simulink model "controller_PRM_BFS_smooth"  (R2023b)
settings: Solver=VariableStepAuto  StartTime=0.0  StopTime=200  RelTol=1e-3
StopFcn:
  | %plot_trajectory(out.x.Data(:,1), out.y.Data(:,1), 'x [m]', 'y [m]', fullfile('C:\Users\paolo\OneDrive - MSFT\Documenti\Personali\Scuola\università\magistrale\2° ANNO\Secondo Semestre\FSR\Project\Software\Images\Paper\Chapter_4_simulation\smooth\simulink', 'current_trajectory.pdf'));
  | %plot_trajectory(out.x_d.Data(1,:), out.y_d.Data(1,:), '$x_d$ [m]', '$y_d$ [m]', fullfile('C:\Users\paolo\OneDrive - MSFT\Documenti\Personali\Scuola\università\magistrale\2° ANNO\Secondo Semestre\FSR\Project\Software\Images\Paper\Chapter_4_simulation\smooth\simulink', 'desidered_trajectory.pdf'));
  | %plot_velocity(out.v.Time, out.omega.Time, out.v.Data(:,1), out.omega.Data(:,1), 'time [s]', 'v [m/s]', '$\omega$ [rad/s]', fullfile('C:\Users\paolo\OneDrive - MSFT\Documenti\Personali\Scuola\università\magistrale\2° ANNO\Secondo Semestre\FSR\Project\Software\Images\Paper\Chapter_4_simulation\smooth\simulink', 'velocity.pdf'));
  | %plot_error(out.x.Time, out.x_d.Data(1,:), out.x.Data(:,1), 'time [s]', '$e_x$ [m]', fullfile('C:\Users\paolo\OneDrive - MSFT\Documenti\Personali\Scuola\università\magistrale\2° ANNO\Secondo Semestre\FSR\Project\Software\Images\Paper\Chapter_4_simulation\smooth\simulink', 'error_x.pdf'));
  | %plot_error(out.y.Time, out.y_d.Data(1,:), out.y.Data(:,1), 'time [s]', '$e_y$ [m]', fullfile('C:\Users\paolo\OneDrive - MSFT\Documenti\Personali\Scuola\università\magistrale\2° ANNO\Secondo Semestre\FSR\Project\Software\Images\Paper\Chapter_4_simulation\smooth\simulink', 'error_y.pdf'));
  | %plot_error(out.theta.Time, out.theta_d.Data(1,:), out.theta.Data(:,1), 'time [s]', '$e_{\theta}$ [rad]', fullfile('C:\Users\paolo\OneDrive - MSFT\Documenti\Personali\Scuola\università\magistrale\2° ANNO\Secondo Semestre\FSR\Project\Software\Images\Paper\Chapter_4_simulation\smooth\simulink', 'error_theta.pdf'));
  | %plot_error(out.phi.Time, out.phi_d.Data(1,:), out.phi.Data(:,1), 'time [s]', '$e_{\phi}$ [rad]', fullfile('C:\Users\paolo\OneDrive - MSFT\Documenti\Personali\Scuola\università\magistrale\2° ANNO\Secondo Semestre\FSR\Project\Software\Images\Paper\Chapter_4_simulation\smooth\simulink', 'error_phi.pdf'));
libraries: robotmobilelib x1
settings Model: LastModifiedBy=paolo
settings ModelReferenceCC: EnableRefExpFcnMdlSchedulingChecks=on

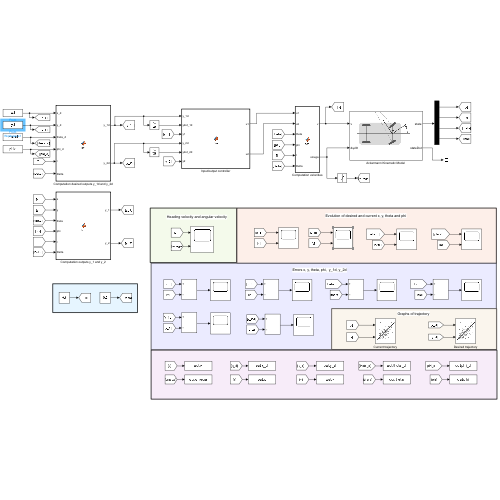
[thumbnail: Simulink's stored preview of the top-level diagram]
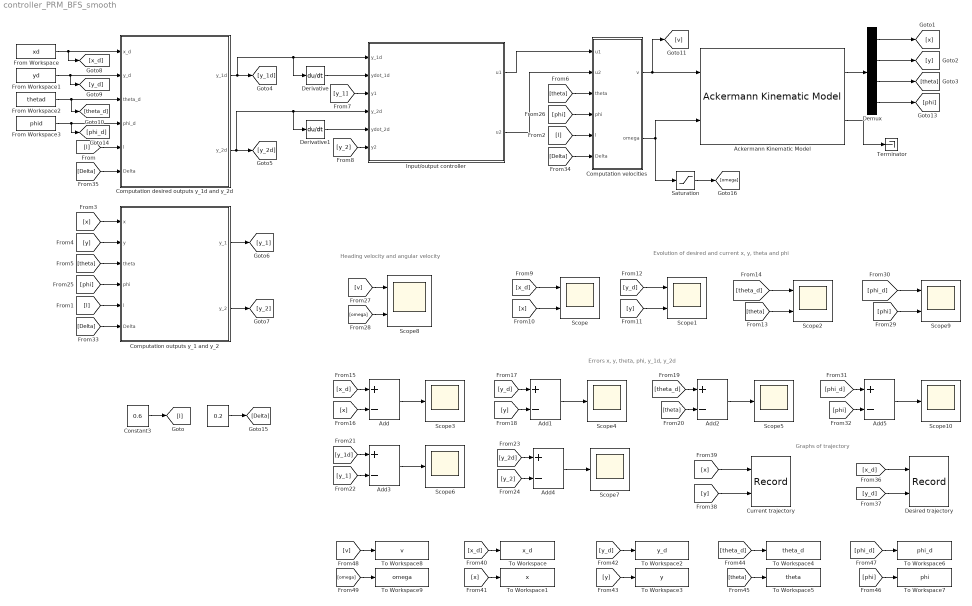
== system controller_PRM_BFS_smooth ==
  note: Errors x, y, theta, phi, y_1d, y_2d
  note: Evolution of desired and current x, y, theta and phi
  note: Heading velocity and angular velocity
  note: Graphs of trajectory
  " " : Constant  Value=0.2
  "Ackermann Kinematic Model " : robotmobilelib/Ackermann Kinematic Model  WheelBase=0.6  VehicleSpeedRange=[-3 3]  MaxSteeringAngle=pi/4  InitialState=q0  SimulateUsing=Interpreted execution
  Add{,1..5} (6 alike) : Sum  Inputs=+-
  Computation desired outputs y_1d and y_2d : MATLAB Function  TreatAsAtomicUnit=on
  Computation outputs y_1 and y_2 : MATLAB Function  TreatAsAtomicUnit=on
  Computation velocities : MATLAB Function  TreatAsAtomicUnit=on
  Constant3 : Constant  Value=0.6
  Current trajectory : Record  FileSettingsInternal="{\"entries\":[{\"content\":{\"excelSettings\":{\"content\":{},\"type\":\"Streamout.ExcelSettings\"}},\"type\":\"Streamout.FileSettingStorage\",\"uuid\":\"\"}],\"packageUris\":[\"http:\\/\\/schema.mathworks.com\\/mf0\\/streamout_blocks\\/R2020a\"],\"version\":\"1.0\"}"  Layout=[1 1]  SignalsInternal="{\"entries\":[{\"content\":{\"signals\":[{\"content\":{\"blockPath\":[],\"dimensions\":[1],\"domain\":\"\",\"lineColor\":\"#edb120\",\"plots\":[1],\"port\":1,\"signalID\":32,\"signalName\":\"From39\"},\"type\":\"RecordBlkView.Signal\",\"uuid\":\"\"},{\"content\":{\"blockPath\":[],\"dimensions\":[1],\"domain\":\"\",\"lineColor\":\"#7e2f8e\",\"plots\":[1],\"port\":2,\"signalID\":35,\"signalName\":\"From38\"},\"type\":\"RecordBlkView.Signal\",\"uuid\":\"\"}]},\"type\":\"RecordBlkView.InputSignals\",\"uuid\":\"\"}],\"packageUris\":[\"http:\\/\\/schema.mathworks.com\\/mf0\\/streamout_blocks\\/R2020a\"],\"version\":\"1.0\"}"  VisualizationBindings="{\"xyplotplugin\":{\"info\":[{\"series\":[{\"bindingParametersList\":[{\"parameter\":\"X-Axis\",\"signalID\":32,\"signalName\":\"From39\"},{\"parameter\":\"Y-Axis\",\"signalID\":35,\"signalName\":\"From38\"}],\"seriesID\":35682}],\"subplotID\":1}]}}"  CompatibilityTag=XY
  Demux : Demux
  Derivative : Derivative
  Derivative1 : Derivative
  Desired trajectory : Record  FileSettingsInternal="{\"entries\":[{\"content\":{\"excelSettings\":{\"content\":{},\"type\":\"Streamout.ExcelSettings\"}},\"type\":\"Streamout.FileSettingStorage\",\"uuid\":\"\"}],\"packageUris\":[\"http:\\/\\/schema.mathworks.com\\/mf0\\/streamout_blocks\\/R2020a\"],\"version\":\"1.0\"}"  Layout=[1 1]  SignalsInternal="{\"entries\":[{\"content\":{\"signals\":[{\"content\":{\"blockPath\":[],\"dimensions\":[1,1],\"domain\":\"\",\"lineColor\":\"#77ac30\",\"plots\":[1],\"port\":1,\"signalID\":24,\"signalName\":\"From36\"},\"type\":\"RecordBlkView.Signal\",\"uuid\":\"\"},{\"content\":{\"blockPath\":[],\"dimensions\":[1,1],\"domain\":\"\",\"lineColor\":\"#4dbeee\",\"plots\":[1],\"port\":2,\"signalID\":27,\"signalName\":\"From37\"},\"type\":\"RecordBlkView.Signal\",\"uuid\":\"\"}]},\"type\":\"RecordBlkView.InputSignals\",\"uuid\":\"\"}],\"packageUris\":[\"http:\\/\\/schema.mathworks.com\\/mf0\\/streamout_blocks\\/R2020a\"],\"version\":\"1.0\"}"  VisualizationBindings="{\"xyplotplugin\":{\"info\":[{\"series\":[{\"bindingParametersList\":[{\"parameter\":\"X-Axis\",\"signalID\":24,\"signalName\":\"From36\"},{\"parameter\":\"Y-Axis\",\"signalID\":27,\"signalName\":\"From37\"}],\"seriesID\":37876}],\"subplotID\":1}]}}"  CompatibilityTag=XY
  From Workspace : FromWorkspace  VariableName=xd
  From Workspace1 : FromWorkspace  VariableName=yd
  From Workspace2 : FromWorkspace  VariableName=thetad
  From Workspace3 : FromWorkspace  VariableName=phid
  Input/output controller : MATLAB Function  TreatAsAtomicUnit=on
  Saturation : Saturate  UpperLimit=0.43  LowerLimit=-0.43  ZeroCross=off
  Scope{,1..2,8..9} (5 alike) : Scope  NumInputPorts=2
  Scope{3..7,10} (6 alike) : Scope
  Terminator : Terminator
  To Workspace : ToWorkspace  VariableName=x_d  SaveFormat=Timeseries  SampleTime=-1
  To Workspace1 : ToWorkspace  VariableName=x  SaveFormat=Timeseries  SampleTime=-1
  To Workspace2 : ToWorkspace  VariableName=y_d  SaveFormat=Timeseries  SampleTime=-1
  To Workspace3 : ToWorkspace  VariableName=y  SaveFormat=Timeseries  SampleTime=-1
  To Workspace4 : ToWorkspace  VariableName=theta_d  SaveFormat=Timeseries  SampleTime=-1
  To Workspace5 : ToWorkspace  VariableName=theta  SaveFormat=Timeseries  SampleTime=-1
  To Workspace6 : ToWorkspace  VariableName=phi_d  SaveFormat=Timeseries  SampleTime=-1
  To Workspace7 : ToWorkspace  VariableName=phi  SaveFormat=Timeseries  SampleTime=-1
  To Workspace8 : ToWorkspace  VariableName=v  SaveFormat=Timeseries  SampleTime=-1
  To Workspace9 : ToWorkspace  VariableName=omega  SaveFormat=Timeseries  SampleTime=-1
  wires:
  Computation velocities/2(omega) -> Saturation/1, "Ackermann Kinematic Model "/2
  From Workspace/1 -> Computation desired outputs y_1d and y_2d/1(x_d), [x_d]
  From Workspace1/1 -> [y_d], Computation desired outputs y_1d and y_2d/2(y_d)
  From Workspace2/1 -> [theta_d], Computation desired outputs y_1d and y_2d/3(theta_d)
  Constant3/1 -> [l]
  [l] -> Computation desired outputs y_1d and y_2d/5(l)
  Computation desired outputs y_1d and y_2d/1(y_1d) -> [y_1d], Input/output controller/1(y_1d), Derivative/1
  Input/output controller/1(u1) -> Computation velocities/1(u1)
  Input/output controller/2(u2) -> Computation velocities/2(u2)
  [l] -> Computation outputs y_1 and y_2/5(l)
  [l] -> Computation velocities/5(l)
  Demux/3 -> [theta]
  [x] -> Computation outputs y_1 and y_2/1(x)
  [y] -> Computation outputs y_1 and y_2/2(y)
  [theta] -> Computation outputs y_1 and y_2/3(theta)
  [theta] -> Computation velocities/3(theta)
  Computation desired outputs y_1d and y_2d/2(y_2d) -> [y_2d], Input/output controller/4(y_2d), Derivative1/1
  Computation outputs y_1 and y_2/1(y_1) -> [y_1]
  Computation outputs y_1 and y_2/2(y_2) -> [y_2]
  [y_1] -> Input/output controller/3(y1)
  [y_2] -> Input/output controller/6(y2)
  [x_d] -> Scope/1
  [x] -> Scope/2
  [y_d] -> Scope1/1
  [y] -> Scope1/2
  [theta_d] -> Scope2/1
  [theta] -> Scope2/2
  [x_d] -> Add/1
  [x] -> Add/2
  Add/1 -> Scope3/1
  [y_d] -> Add1/1
  [y] -> Add1/2
  Add1/1 -> Scope4/1
  [theta_d] -> Add2/1
  [theta] -> Add2/2
  Add2/1 -> Scope5/1
  Add3/1 -> Scope6/1
  [y_1] -> Add3/2
  [y_1d] -> Add3/1
  Add4/1 -> Scope7/1
  [y_2] -> Add4/2
  [y_2d] -> Add4/1
  Demux/1 -> [x]
  Demux/2 -> [y]
  Computation velocities/1(v) -> [v], "Ackermann Kinematic Model "/1
  [v] -> Scope8/1
  [omega] -> Scope8/2
  Demux/4 -> [phi]
  [phi] -> Computation outputs y_1 and y_2/4(phi)
  From Workspace3/1 -> Computation desired outputs y_1d and y_2d/4(phi_d), [phi_d]
  [phi] -> Computation velocities/4(phi)
  "Ackermann Kinematic Model "/1 -> Demux/1
  "Ackermann Kinematic Model "/2 -> Terminator/1
  [phi_d] -> Scope9/1
  [phi] -> Scope9/2
  Add5/1 -> Scope10/1
  [phi_d] -> Add5/1
  [phi] -> Add5/2
  Derivative1/1 -> Input/output controller/5(ydot_2d)
  Derivative/1 -> Input/output controller/2(ydot_1d)
  " "/1 -> [Delta]
  [Delta] -> Computation outputs y_1 and y_2/6(Delta)
  [Delta] -> Computation velocities/6(Delta)
  [Delta] -> Computation desired outputs y_1d and y_2d/6(Delta)
  [y_d] -> Desired trajectory/2
  [x_d] -> Desired trajectory/1
  [x] -> Current trajectory/1
  [y] -> Current trajectory/2
  Saturation/1 -> [omega]
  [x_d] -> To Workspace/1
  [x] -> To Workspace1/1
  [y_d] -> To Workspace2/1
  [y] -> To Workspace3/1
  [theta_d] -> To Workspace4/1
  [theta] -> To Workspace5/1
  [phi_d] -> To Workspace6/1
  [phi] -> To Workspace7/1
  [omega] -> To Workspace9/1
  [v] -> To Workspace8/1

== matlab function controller_PRM_BFS_smooth/Computation desired outputs y_1d and y_2d ==
  data: x_d input; y_1d output; y_d input; theta_d input; phi_d input; y_2d output; l input; Delta input
function [y_1d, y_2d]  = fcn(x_d, y_d, theta_d, phi_d, l, Delta)

y_1d = x_d+l*cos(theta_d)+Delta*cos(theta_d+phi_d);
y_2d = y_d+l*sin(theta_d)+Delta*sin(theta_d+phi_d);
 
end

== matlab function controller_PRM_BFS_smooth/Computation velocities ==
  data: u1 input; v output; omega output; u2 input; theta input; phi input; l input; Delta input
function [v, omega] = fcn(u1, u2, theta, phi, l, Delta)

T = [cos(theta)-tan(phi)*(sin(theta)+(Delta*sin(theta+phi))/l) -Delta*sin(theta+phi);
     sin(theta)+tan(phi)*(cos(theta)+(Delta*cos(theta+phi))/l) +Delta*cos(theta+phi)];

Tinv = inv(T);

v = Tinv(1,:)*[u1; u2];
omega = Tinv(2,:)*[u1; u2];


end

== matlab function controller_PRM_BFS_smooth/Input//output controller ==
  data: y_1d input; u1 output; ydot_1d input; y1 input; y_2d input; ydot_2d input; y2 input; u2 output
function [u1, u2] = fcn(y_1d, ydot_1d, y1, y_2d, ydot_2d, y2)

k1 = 5; 
k2 = 5; 

u1 = ydot_1d+k1*(y_1d-y1);
u2 = ydot_2d+k2*(y_2d-y2);

end

== matlab function controller_PRM_BFS_smooth/Computation outputs y_1 and y_2 ==
  data: x input; y_1 output; y input; theta input; phi input; y_2 output; l input; Delta input
function [y_1, y_2]  = fcn(x, y, theta, phi, l, Delta)

y_1 = x+l*cos(theta)+Delta*cos(theta+phi);
y_2 = y+l*sin(theta)+Delta*sin(theta+phi);

end
